simulink model "DC_Motor"  (R2025b)
settings: Solver=VariableStepAuto  StartTime=0.0  StopTime=10.0  RelTol=1e-3
undefined symbols (not defined in the file): b, J, K, L, R

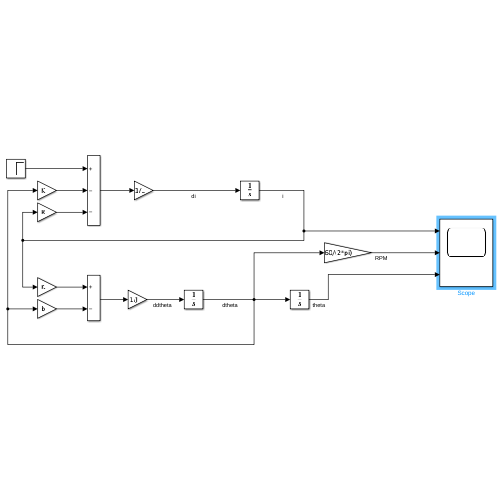
[thumbnail: Simulink's stored preview of the top-level diagram]
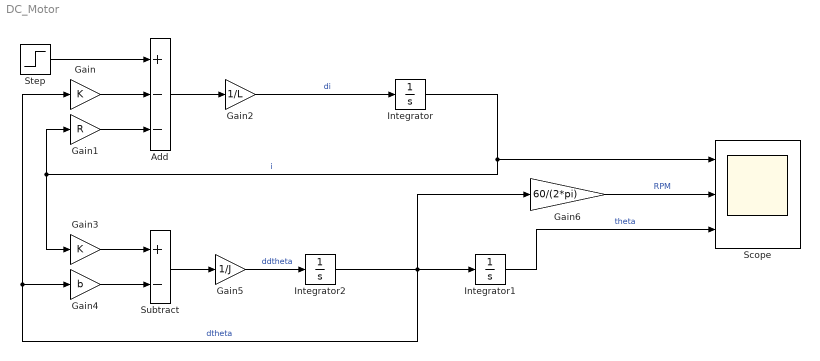
== system DC_Motor ==
  Add : Sum  Inputs=+--
  Gain : Gain  Gain=K
  Gain1 : Gain  Gain=R
  Gain2 : Gain  Gain=1/L
  Gain3 : Gain  Gain=K
  Gain4 : Gain  Gain=b
  Gain5 : Gain  Gain=1/J
  Gain6 : Gain  Gain=60/(2*pi)
  Integrator : Integrator
  Integrator1 : Integrator
  Integrator2 : Integrator
  Scope : Scope  NumInputPorts=3
      settings: ActiveDisplayYMinimum=-16.872185398903742  ActiveDisplayYMaximum=52.7417890605043
  Step : Step  SampleTime=0
  Subtract : Sum  Inputs=+-
  wires:
  Integrator1/1 -> Scope/3  "theta"
  Gain4/1 -> Subtract/2
  Integrator/1 -> Gain1/1, Gain3/1, Scope/1  "i"
  Step/1 -> Add/1
  Gain3/1 -> Subtract/1
  Gain2/1 -> Integrator/1  "di"
  Subtract/1 -> Gain5/1
  Gain6/1 -> Scope/2  "RPM"
  Integrator2/1 -> Gain6/1, Gain4/1, Gain/1, Integrator1/1  "dtheta"
  Gain1/1 -> Add/3
  Add/1 -> Gain2/1
  Gain5/1 -> Integrator2/1  "ddtheta"
  Gain/1 -> Add/2
